simulink library "smoothTransition"  (R2018a)
settings: Solver=VariableStepAuto  StartTime=0.0  StopTime=10.0  RelTol=1e-3
undefined symbols (not defined in the file or in its folder): ctrl, iterationPhase_enum, plant
libraries: simulink x2, controllerComponents x1, determineIterationPhase_ul x1, determineSimulationPhase_ul x1, findClosestPointOnPath_cl x1, getTargetPoint x1, ILCUpdate x1, PerformanceIndex x1, rudderController x1, stabilizerController_ul x1, tetherSpeedController x1, wingController x1
settings Model: Creator=mitch  LastModifiedBy=M.Cobb

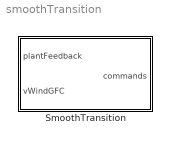
== system smoothTransition ==
  SmoothTransition : Subsystem  VariantControl=variantSmoothTransition

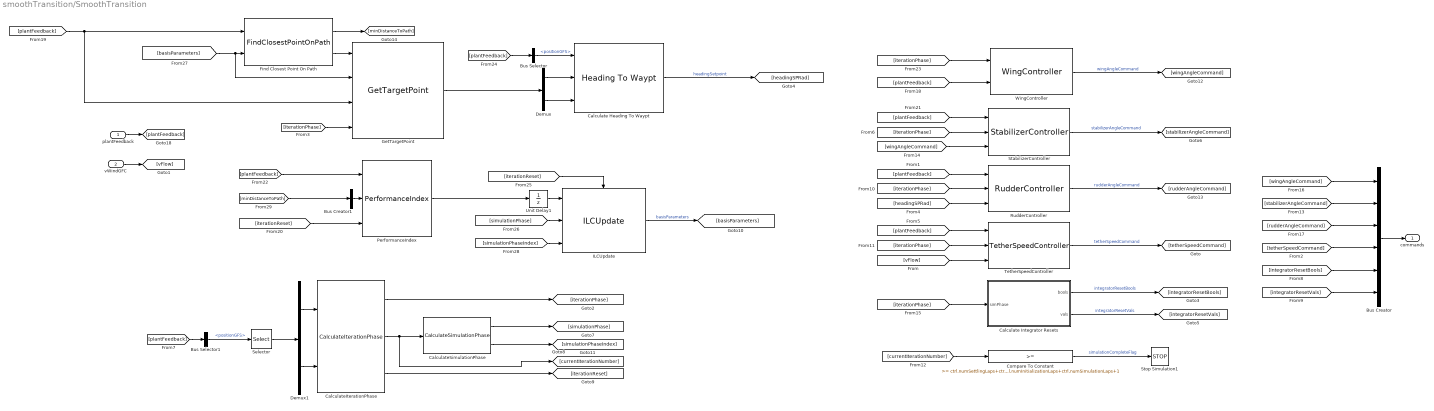
== system smoothTransition/SmoothTransition ==
  plantFeedback : Inport  OutDataTypeStr=Bus: busPlantFeedback
  vWindGFC : Inport  Port=2
  Bus Creator : BusCreator  Inputs=6  OutDataTypeStr=Bus: busControllerOutput
  Bus Creator1 : BusCreator  Inputs=1
  Bus Selector : BusSelector  OutputSignals=positionGFS
  Bus Selector1 : BusSelector  OutputSignals=positionGFS
  Calculate Heading To Waypt : controllerComponents/Heading To Waypt
  Calculate Integrator Resets : Subsystem
  CalculateIterationPhase : determineIterationPhase_ul/CalculateIterationPhase
  CalculateSimulationPhase : determineSimulationPhase_ul/CalculateSimulationPhase
  Compare To Constant : simulink/Logic and Bit Operations/Compare To Constant  relop=>=  const=ctrl.numSettlingLaps+ctrl.numInitializationLaps+ctrl.numSimulationLaps+1  OutDataTypeStr=boolean
  Demux : Demux  Outputs=2
  Demux1 : Demux  Outputs=2
  Find Closest Point On Path : findClosestPointOnPath_cl/FindClosestPointOnPath
  GetTargetPoint : getTargetPoint/GetTargetPoint
  ILCUpdate : ILCUpdate/ILCUpdate
  PerformanceIndex : PerformanceIndex/PerformanceIndex
  RudderController : rudderController/RudderController
  Selector : Selector  InputPortWidth=3  IndexOptions=Index vector (dialog)  Indices=[1 2]  OutputSizes=1
  StabilizerController : stabilizerController_ul/StabilizerController
  Stop Simulation1 : Stop
  TetherSpeedController : tetherSpeedController/TetherSpeedController
  Unit Delay1 : UnitDelay  SampleTime=-1
  WingController : wingController/WingController
  commands : Outport  OutDataTypeStr=Bus: busControllerOutput
  wires:
  [minDistanceToPath] -> Bus Creator1/1
  Bus Creator1/1 -> PerformanceIndex/2
  Unit Delay1/1 -> ILCUpdate/1
  [wingAngleCommand] -> StabilizerController/3
  [plantFeedback] -> StabilizerController/1
  [iterationPhase] -> StabilizerController/2
  [iterationPhase] -> RudderController/2
  [headingSPRad] -> RudderController/3
  [plantFeedback] -> RudderController/1
  [stabilizerAngleCommand] -> Bus Creator/2
  StabilizerController/1 -> [stabilizerAngleCommand]  "stabilizerAngleCommand"
  [wingAngleCommand] -> Bus Creator/1
  [rudderAngleCommand] -> Bus Creator/3
  [tetherSpeedCommand] -> Bus Creator/4
  [integratorResetBools] -> Bus Creator/5
  [integratorResetVals] -> Bus Creator/6
  [iterationPhase] -> TetherSpeedController/2
  [plantFeedback] -> TetherSpeedController/1
  [vFlow] -> TetherSpeedController/3
  Calculate Integrator Resets/2(vals) -> [integratorResetVals]  "integratorResetVals"
  Calculate Integrator Resets/1(bools) -> [integratorResetBools]  "integratorResetBools"
  [iterationPhase] -> Calculate Integrator Resets/1(simPhase)
  [iterationPhase] -> WingController/1
  WingController/1 -> [wingAngleCommand]  "wingAngleCommand"
  [plantFeedback] -> WingController/2
  TetherSpeedController/1 -> [tetherSpeedCommand]  "tetherSpeedCommand"
  RudderController/1 -> [rudderAngleCommand]  "rudderAngleCommand"
  Calculate Heading To Waypt/1 -> [headingSPRad]  "headingSetpoint"
  Compare To Constant/1 -> Stop Simulation1/1  "simulationCompleteFlag"
  [currentIterationNumber] -> Compare To Constant/1
  Bus Creator/1 -> commands/1
  vWindGFC/1 -> [vFlow]
  plantFeedback/1 -> [plantFeedback]
  [plantFeedback] -> GetTargetPoint/3, Find Closest Point On Path/1
  Find Closest Point On Path/2 -> GetTargetPoint/1
  [basisParameters] -> GetTargetPoint/2, Find Closest Point On Path/2
  Find Closest Point On Path/1 -> [minDistanceToPath]
  [plantFeedback] -> Bus Selector/1
  Bus Selector/1 -> Calculate Heading To Waypt/1  "<positionGFS>"
  Demux/1 -> Calculate Heading To Waypt/2
  Demux/2 -> Calculate Heading To Waypt/3
  CalculateIterationPhase/2 -> [currentIterationNumber], CalculateSimulationPhase/1
  [plantFeedback] -> Bus Selector1/1
  Bus Selector1/1 -> Selector/1  "<positionGFS>"
  Demux1/1 -> CalculateIterationPhase/1
  Demux1/2 -> CalculateIterationPhase/2
  Selector/1 -> Demux1/1
  CalculateSimulationPhase/1 -> [simulationPhase]
  CalculateIterationPhase/1 -> [iterationPhase]
  GetTargetPoint/1 -> Demux/1
  [iterationPhase] -> GetTargetPoint/4
  CalculateIterationPhase/3 -> [iterationReset]
  [iterationReset] -> PerformanceIndex/3
  [plantFeedback] -> PerformanceIndex/1
  PerformanceIndex/1 -> Unit Delay1/1
  [iterationReset] -> ILCUpdate/Trigger
  [simulationPhase] -> ILCUpdate/2
  ILCUpdate/1 -> [basisParameters]  "basisParameters"
  CalculateSimulationPhase/2 -> [simulationPhaseIndex]
  [simulationPhaseIndex] -> ILCUpdate/3

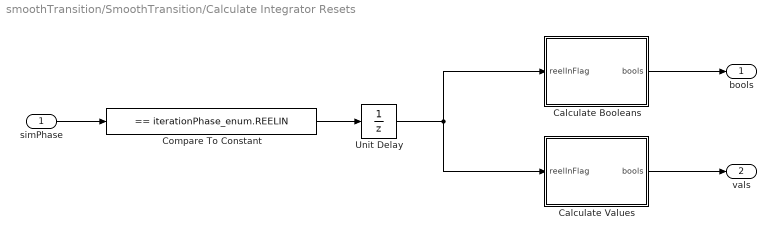
== system smoothTransition/SmoothTransition/Calculate Integrator Resets ==
  simPhase : Inport
  Calculate Booleans : Subsystem
  Calculate Values : Subsystem
  Compare To Constant : simulink/Logic and Bit Operations/Compare To Constant  relop===  const=iterationPhase_enum.REELIN  OutDataTypeStr=boolean
  Unit Delay : UnitDelay  InitialCondition=false  SampleTime=-1
  bools : Outport
  vals : Outport  Port=2
  wires:
  Calculate Values/1(bools) -> vals/1
  Calculate Booleans/1(bools) -> bools/1
  Compare To Constant/1 -> Unit Delay/1
  simPhase/1 -> Compare To Constant/1
  Unit Delay/1 -> Calculate Values/1(reelInFlag), Calculate Booleans/1(reelInFlag)

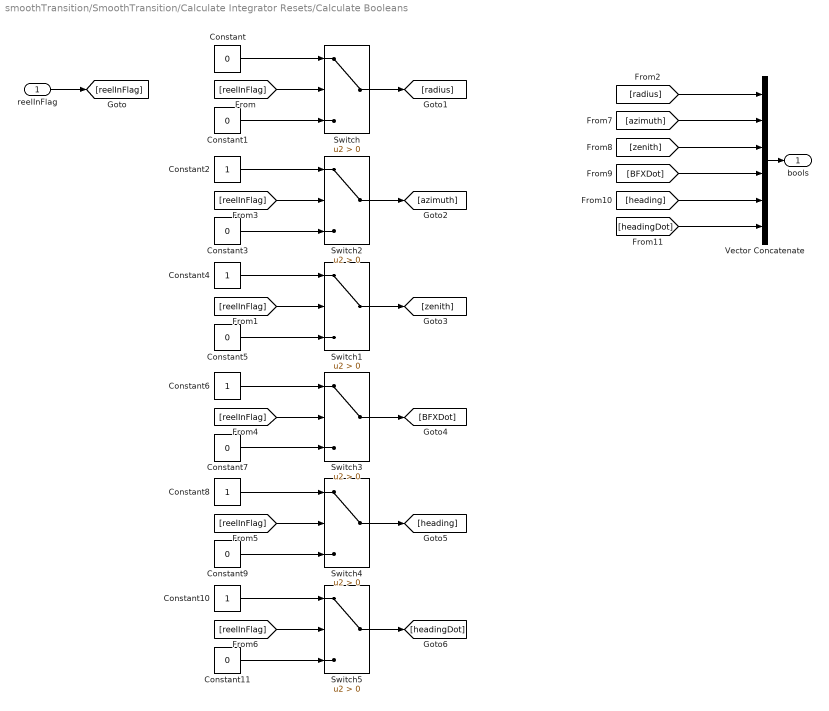
== system smoothTransition/SmoothTransition/Calculate Integrator Resets/Calculate Booleans ==
  reelInFlag : Inport
  Constant{,1,3,5,7,9,11} (7 alike) : Constant  Value=0  OutDataTypeStr=boolean
  Constant{2,4,6,8,10} (5 alike) : Constant  OutDataTypeStr=boolean
  Switch{,1..5} (6 alike) : Switch  Criteria=u2 > Threshold
  Vector Concatenate : Concatenate  NumInputs=6
  bools : Outport
  wires:
  reelInFlag/1 -> [reelInFlag]
  [reelInFlag] -> Switch2/2
  Switch2/1 -> [azimuth]
  Constant3/1 -> Switch2/3
  Constant2/1 -> Switch2/1
  Vector Concatenate/1 -> bools/1
  Switch3/1 -> [BFXDot]
  Constant6/1 -> Switch3/1
  [reelInFlag] -> Switch3/2
  Constant7/1 -> Switch3/3
  Constant1/1 -> Switch/3
  Switch/1 -> [radius]
  Constant/1 -> Switch/1
  Constant11/1 -> Switch5/3
  Constant10/1 -> Switch5/1
  Switch5/1 -> [headingDot]
  [reelInFlag] -> Switch5/2
  Switch1/1 -> [zenith]
  [reelInFlag] -> Switch/2
  [reelInFlag] -> Switch1/2
  Constant4/1 -> Switch1/1
  Constant5/1 -> Switch1/3
  [reelInFlag] -> Switch4/2
  Constant9/1 -> Switch4/3
  Switch4/1 -> [heading]
  Constant8/1 -> Switch4/1
  [azimuth] -> Vector Concatenate/2
  [zenith] -> Vector Concatenate/3
  [BFXDot] -> Vector Concatenate/4
  [heading] -> Vector Concatenate/5
  [headingDot] -> Vector Concatenate/6
  [radius] -> Vector Concatenate/1

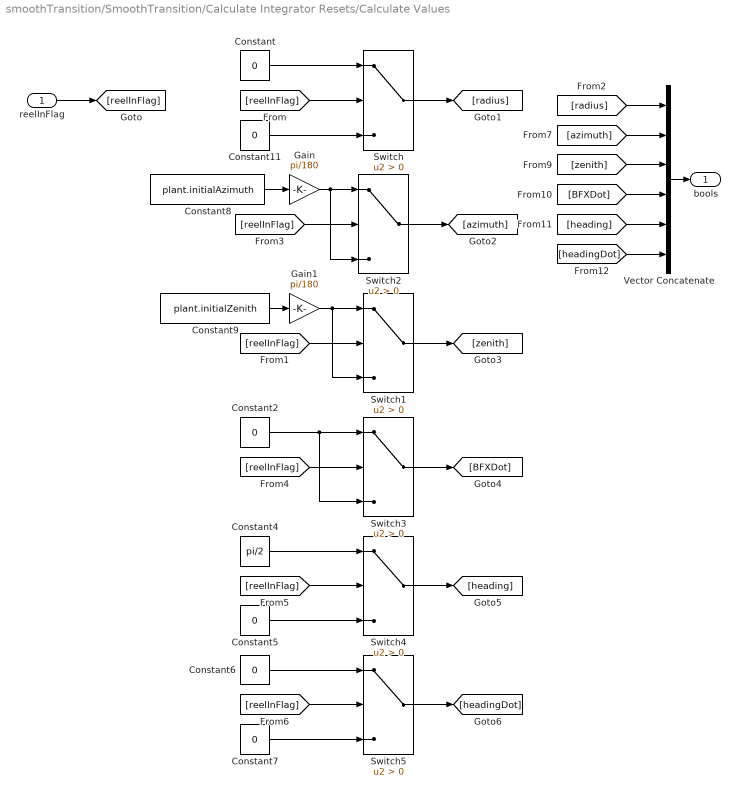
== system smoothTransition/SmoothTransition/Calculate Integrator Resets/Calculate Values ==
  reelInFlag : Inport
  Constant{,2,5..7,11} (6 alike) : Constant  Value=0  OutDataTypeStr=double
  Constant4 : Constant  Value=pi/2  OutDataTypeStr=double
  Constant8 : Constant  Value=plant.initialAzimuth  OutDataTypeStr=double
  Constant9 : Constant  Value=plant.initialZenith  OutDataTypeStr=double
  Gain : Gain  Gain=pi/180
  Gain1 : Gain  Gain=pi/180
  Switch{,1..5} (6 alike) : Switch  Criteria=u2 > Threshold
  Vector Concatenate : Concatenate  NumInputs=6
  bools : Outport
  wires:
  reelInFlag/1 -> [reelInFlag]
  [headingDot] -> Vector Concatenate/6
  [reelInFlag] -> Switch2/2
  Switch2/1 -> [azimuth]
  Gain/1 -> Switch2/1, Switch2/3
  Constant8/1 -> Gain/1
  [heading] -> Vector Concatenate/5
  [zenith] -> Vector Concatenate/3
  [azimuth] -> Vector Concatenate/2
  Vector Concatenate/1 -> bools/1
  Switch3/1 -> [BFXDot]
  [reelInFlag] -> Switch3/2
  Constant2/1 -> Switch3/1, Switch3/3
  Constant11/1 -> Switch/3
  Switch/1 -> [radius]
  [BFXDot] -> Vector Concatenate/4
  Constant/1 -> Switch/1
  Constant7/1 -> Switch5/3
  Constant6/1 -> Switch5/1
  Switch5/1 -> [headingDot]
  [reelInFlag] -> Switch5/2
  [radius] -> Vector Concatenate/1
  Switch1/1 -> [zenith]
  [reelInFlag] -> Switch/2
  [reelInFlag] -> Switch1/2
  Constant9/1 -> Gain1/1
  Gain1/1 -> Switch1/1, Switch1/3
  [reelInFlag] -> Switch4/2
  Constant5/1 -> Switch4/3
  Switch4/1 -> [heading]
  Constant4/1 -> Switch4/1
